simulink model "prelab1_1"  (R2025b)
settings: Solver=VariableStepAuto  StartTime=0.0  StopTime=30  RelTol=1e-7

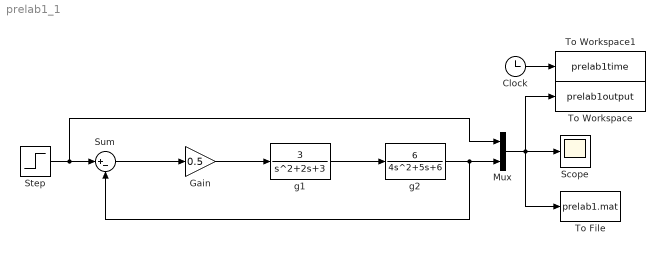
== system prelab1_1 ==
  Clock : Clock
  Gain : Gain  Gain=0.5
  Mux : Mux  Inputs=2
  Scope : Scope
      settings: ActiveDisplayYMinimum=0.1253042056430147  ActiveDisplayYMaximum=0.60252680812229065
  Step : Step  Time=0  SampleTime=0
  Sum : Sum  Inputs=|+-
  To File : ToFile  Filename=prelab1.mat  SaveFormat=Timeseries
  To Workspace : ToWorkspace  VariableName=prelab1output  SampleTime=-1
  To Workspace1 : ToWorkspace  VariableName=prelab1time  SampleTime=-1
  g1 : TransferFcn  Numerator=[3]  Denominator=[1 2 3]
  g2 : TransferFcn  Numerator=[6]  Denominator=[4 5 6]
  wires:
  Sum/1 -> Gain/1
  Gain/1 -> g1/1
  g1/1 -> g2/1
  g2/1 -> Sum/2, Mux/2
  Step/1 -> Mux/1, Sum/1
  Mux/1 -> To File/1, To Workspace/1, Scope/1
  Clock/1 -> To Workspace1/1
